simulink model "actuador"  (R2017b)
settings: Solver=FixedStepAuto  StartTime=0.0  StopTime=tmax  RelTol=1e-3
undefined symbols (not defined in the file): Beq, f_pwm, Im_max, Jeq, Kdp, Kdv, Kip, Kiv, Km, Kpp, Kpv, Lm, Rm, Vin_pwm, Vout_pwm
libraries: simulink x4
settings Model: Creator=JesusC  LastModifiedBy=JesusC

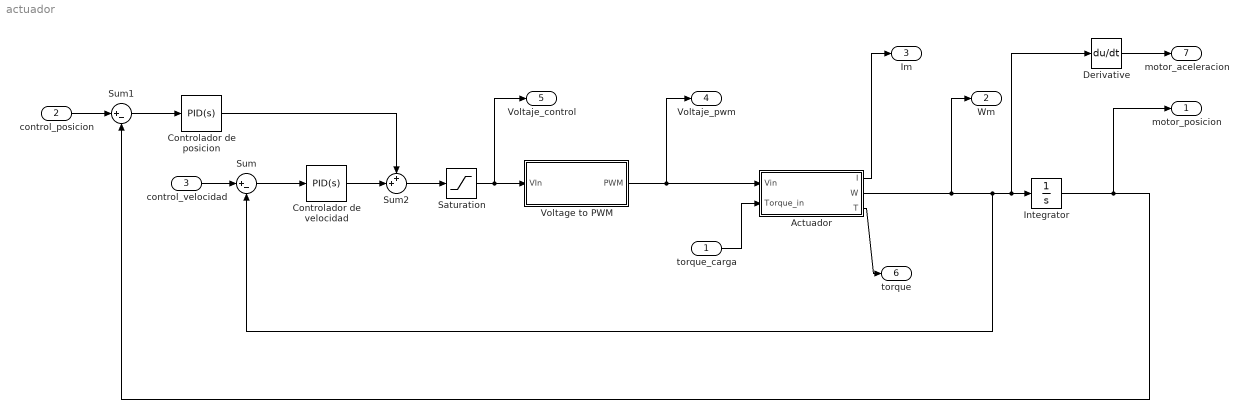
== system actuador ==
  torque_carga : Inport
  control_posicion : Inport  Port=2
  control_velocidad : Inport  Port=3
  "Actuador " : Subsystem
  Controlador de posicion : simulink/Continuous/PID Controller  Controller=PID  TimeDomain=Continuous-time  SampleTime=-1  IntegratorMethod=Forward Euler  FilterMethod=Forward Euler  Form=Parallel  UseFilter=on  ControllerParametersSource=internal  P=Kpp  I=Kip  D=Kdp  N=10000  InitialConditionSource=internal  InitialConditionForIntegrator=0  InitialConditionForFilter=0  ExternalReset=none  LimitOutput=off  UpperSaturationLimit=inf  LowerSaturationLimit=-inf  LinearizeAsGain=on  AntiWindupMode=none  Kb=1  TrackingMode=off  Kt=1  PParamMin=[]  PParamMax=[]  IParamMin=[]  IParamMax=[]  DParamMin=[]  DParamMax=[]  NParamMin=[]  NParamMax=[]  KbParamMin=[]  KbParamMax=[]  KtParamMin=[]  KtParamMax=[]  POutMin=[]  POutMax=[]  IOutMin=[]  IOutMax=[]  DOutMin=[]  DOutMax=[]  NOutMin=[]  NOutMax=[]  KbOutMin=[]  KbOutMax=[]  KtOutMin=[]  KtOutMax=[]  IntegratorOutMin=[]  IntegratorOutMax=[]  FilterOutMin=[]  FilterOutMax=[]  SumOutMin=[]  SumOutMax=[]  SumI1OutMin=[]  SumI1OutMax=[]  SumI2OutMin=[]  SumI2OutMax=[]  SumI3OutMin=[]  SumI3OutMax=[]  SumDOutMin=[]  SumDOutMax=[]  SaturationOutMin=[]  SaturationOutMax=[]  IntegratorContinuousStateAttributes=''  IntegratorStateMustResolveToSignalObject=off  IntegratorRTWStateStorageClass=Auto  FilterContinuousStateAttributes=''  FilterStateMustResolveToSignalObject=off  FilterRTWStateStorageClass=Auto  DifferentiatorICPrevScaledInput=0  DifferentiatorOutMin=[]  DifferentiatorOutMax=[]  InitialConditionSetting=State (most efficient)  FilterDiffOutCoefMin=[]  FilterDiffOutCoefMax=[]  SumDenOutMin=[]  SumDenOutMax=[]  SumNumOutMin=[]  SumNumOutMax=[]  ReciprocalOutMin=[]  ReciprocalOutMax=[]  DivideOutMin=[]  DivideOutMax=[]  TunerSelectOption=Transfer Function Based (PID Tuner App)
  Controlador de velocidad : simulink/Continuous/PID Controller  Controller=PID  TimeDomain=Continuous-time  SampleTime=-1  IntegratorMethod=Forward Euler  FilterMethod=Forward Euler  Form=Parallel  UseFilter=on  ControllerParametersSource=internal  P=Kpv  I=Kiv  D=Kdv  N=10000  InitialConditionSource=internal  InitialConditionForIntegrator=0  InitialConditionForFilter=0  ExternalReset=none  LimitOutput=off  UpperSaturationLimit=inf  LowerSaturationLimit=-inf  LinearizeAsGain=on  AntiWindupMode=none  Kb=1  TrackingMode=off  Kt=1  PParamMin=[]  PParamMax=[]  IParamMin=[]  IParamMax=[]  DParamMin=[]  DParamMax=[]  NParamMin=[]  NParamMax=[]  KbParamMin=[]  KbParamMax=[]  KtParamMin=[]  KtParamMax=[]  POutMin=[]  POutMax=[]  IOutMin=[]  IOutMax=[]  DOutMin=[]  DOutMax=[]  NOutMin=[]  NOutMax=[]  KbOutMin=[]  KbOutMax=[]  KtOutMin=[]  KtOutMax=[]  IntegratorOutMin=[]  IntegratorOutMax=[]  FilterOutMin=[]  FilterOutMax=[]  SumOutMin=[]  SumOutMax=[]  SumI1OutMin=[]  SumI1OutMax=[]  SumI2OutMin=[]  SumI2OutMax=[]  SumI3OutMin=[]  SumI3OutMax=[]  SumDOutMin=[]  SumDOutMax=[]  SaturationOutMin=[]  SaturationOutMax=[]  IntegratorContinuousStateAttributes=''  IntegratorStateMustResolveToSignalObject=off  IntegratorRTWStateStorageClass=Auto  FilterContinuousStateAttributes=''  FilterStateMustResolveToSignalObject=off  FilterRTWStateStorageClass=Auto  DifferentiatorICPrevScaledInput=0  DifferentiatorOutMin=[]  DifferentiatorOutMax=[]  InitialConditionSetting=State (most efficient)  FilterDiffOutCoefMin=[]  FilterDiffOutCoefMax=[]  SumDenOutMin=[]  SumDenOutMax=[]  SumNumOutMin=[]  SumNumOutMax=[]  ReciprocalOutMin=[]  ReciprocalOutMax=[]  DivideOutMin=[]  DivideOutMax=[]  TunerSelectOption=Transfer Function Based (PID Tuner App)
  Derivative : Derivative  CoefficientInTFapproximation=0
  Integrator : Integrator
  Saturation : Saturate  UpperLimit=Vin_pwm  LowerLimit=-Vin_pwm
  Sum : Sum  Inputs=|+-
  Sum1 : Sum  Inputs=|+-
  Sum2 : Sum  Inputs=++|
  Voltage to PWM : Subsystem
  motor_posicion : Outport
  Wm : Outport  Port=2
  Im : Outport  Port=3
  Voltaje_pwm : Outport  Port=4
  Voltaje_control : Outport  Port=5
  torque : Outport  Port=6
  motor_aceleracion : Outport  Port=7
  wires:
  Voltage to PWM/1(PWM) -> Voltaje_pwm/1, "Actuador "/1(Vin)
  "Actuador "/2(W) -> Wm/1, Sum/2, Derivative/1, Integrator/1
  torque_carga/1 -> "Actuador "/2(Torque_in)
  Saturation/1 -> Voltaje_control/1, Voltage to PWM/1(VIn)
  "Actuador "/1(I) -> Im/1
  "Actuador "/3(T) -> torque/1
  Sum/1 -> Controlador de velocidad/1
  Sum1/1 -> Controlador de posicion/1
  Controlador de velocidad/1 -> Sum2/2
  Sum2/1 -> Saturation/1
  Controlador de posicion/1 -> Sum2/1
  control_velocidad/1 -> Sum/1
  control_posicion/1 -> Sum1/1
  Integrator/1 -> motor_posicion/1, Sum1/2
  Derivative/1 -> motor_aceleracion/1

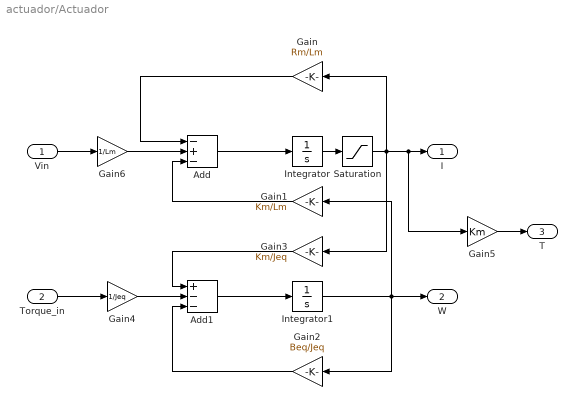
== system actuador/Actuador  ==
  Vin : Inport
  Torque_in : Inport  Port=2
  Add : Sum  Inputs=-+-
  Add1 : Sum  Inputs=+--
  Gain : Gain  Gain=Rm/Lm
  Gain1 : Gain  Gain=Km/Lm
  Gain2 : Gain  Gain=Beq/Jeq
  Gain3 : Gain  Gain=Km/Jeq
  Gain4 : Gain  Gain=1/Jeq
  Gain5 : Gain  Gain=Km
  Gain6 : Gain  Gain=1/Lm
  Integrator : Integrator
  Integrator1 : Integrator
  Saturation : Saturate  UpperLimit=Im_max  LowerLimit=-Im_max
  I : Outport
  W : Outport  Port=2
  T : Outport  Port=3
  wires:
  Integrator/1 -> Saturation/1
  Gain/1 -> Add/1
  Integrator1/1 -> Gain2/1, Gain1/1, W/1
  Gain1/1 -> Add/3
  Add/1 -> Integrator/1
  Add1/1 -> Integrator1/1
  Gain2/1 -> Add1/3
  Gain3/1 -> Add1/1
  Torque_in/1 -> Gain4/1
  Gain4/1 -> Add1/2
  Gain5/1 -> T/1
  Vin/1 -> Gain6/1
  Gain6/1 -> Add/2
  Saturation/1 -> Gain3/1, Gain/1, Gain5/1, I/1

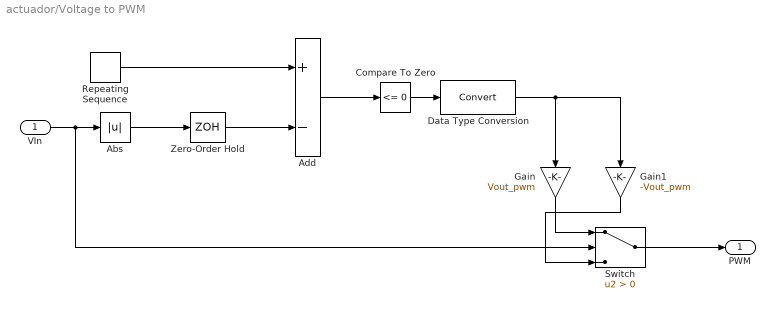
== system actuador/Voltage to PWM ==
  VIn : Inport
  Abs : Abs
  Add : Sum  Inputs=+-
  Compare To Zero : simulink/Logic and Bit Operations/Compare To Zero  relop=<=  OutDataTypeStr=boolean
  Data Type Conversion : DataTypeConversion
  Gain : Gain  Gain=Vout_pwm
  Gain1 : Gain  Gain=-Vout_pwm
  Repeating Sequence : simulink/Sources/Repeating Sequence  rep_seq_t=[0 1/f_pwm]  rep_seq_y=[0 Vin_pwm]
  Switch : Switch  Criteria=u2 > Threshold
  Zero-Order Hold : ZeroOrderHold  SampleTime=-1
  PWM : Outport
  wires:
  Repeating Sequence/1 -> Add/1
  Add/1 -> Compare To Zero/1
  Zero-Order Hold/1 -> Add/2
  Abs/1 -> Zero-Order Hold/1
  VIn/1 -> Switch/2, Abs/1
  Gain/1 -> Switch/1
  Gain1/1 -> Switch/3
  Compare To Zero/1 -> Data Type Conversion/1
  Switch/1 -> PWM/1
  Data Type Conversion/1 -> Gain/1, Gain1/1
